simulink library "pmac"  (R2016b)
settings: Solver=VariableStepAuto  StartTime=0.0  StopTime=10.0  RelTol=1e-3
libraries: hysteresis_rods x1, magnet x1
settings Model: Creator=Sean  LastModifiedBy=Sean

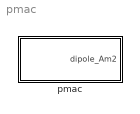
== system pmac ==
  pmac : Subsystem

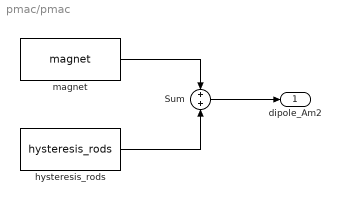
== system pmac/pmac ==
  Sum : Sum
  hysteresis_rods : hysteresis_rods/hysteresis_rods
  magnet : magnet/magnet
  dipole_Am2 : Outport
  wires:
  Sum/1 -> dipole_Am2/1
  magnet/1 -> Sum/1
  hysteresis_rods/1 -> Sum/2
